simulink model "snb_b"  (R2012b)
settings: Solver=FixedStepDiscrete  SolverMode=SingleTasking  StartTime=0.0  StopTime=10000  RelTol=1e-3
undefined symbols (not defined in the file): Down, pfb_coeff_gen_calc, Up, xlipgetpartsetting
libraries: xbsIndex_r4 x14917, casper_library_misc x20, casper_library_communications x8, xps_library x3, casper_library_delays x3
(part 34 of 96)

== system snb_b/unpack_and_reorder/check_timestep_one ==
  note: The timestamp is only allowed to be smaller
      | than or equal to the last timestamp plus one.
  valid : Inport
  time : Inport  Port=2
  AddSub : xbsIndex_r4/AddSub  mode=Addition  use_carryin=off  use_carryout=off  en=off  latency=0  precision=Full  arith_type=Unsigned  n_bits=16  bin_pt=14  quantization=Truncate  overflow=Wrap  dbl_ovrd=off  use_behavioral_HDL=off  hw_selection=Fabric  pipelined=off  block_type=addsub
  Constant1 : xbsIndex_r4/Constant  const=1  gui_display_data_type=Fixed-point  arith_type=Unsigned  n_bits=1  bin_pt=0  preci_type=Single  exp_width=8  frac_width=24  explicit_period=on  period=1  equ=P=C  opselect=C  inp2=PCIN>>17  opr=+  inp1=P  carry=CIN  dbl_ovrd=off  block_type=constant
  Delay1 : xbsIndex_r4/Delay  rst=off  infoeditControl=Selection of Reset will increase slice count due to use of real FFs and instead of SRLs  en=off  latency=1  dbl_ovrd=off  reg_retiming=on  block_type=delay
  Delay2 : xbsIndex_r4/Delay  rst=off  infoeditControl=Selection of Reset will increase slice count due to use of real FFs and instead of SRLs  en=off  latency=1  dbl_ovrd=off  reg_retiming=on  block_type=delay
  Logical : xbsIndex_r4/Logical  logical_function=AND  inputs=2  en=off  latency=1  precision=Full  arith_type=Unsigned  n_bits=16  bin_pt=0  align_bp=on  dbl_ovrd=off  block_type=logical
  Logical1 : xbsIndex_r4/Logical  logical_function=AND  inputs=2  en=off  latency=1  precision=Full  arith_type=Unsigned  n_bits=16  bin_pt=0  align_bp=on  dbl_ovrd=off  block_type=logical
  Logical2 : xbsIndex_r4/Logical  logical_function=OR  inputs=2  en=off  latency=0  precision=Full  arith_type=Unsigned  n_bits=16  bin_pt=0  align_bp=on  dbl_ovrd=off  block_type=logical
  Register4 : xbsIndex_r4/Register  init=0  rst=off  en=on  dbl_ovrd=off  block_type=register
  Relational : xbsIndex_r4/Relational  mode=a>b  en=off  latency=1  dbl_ovrd=off  block_type=relational
  Relational1 : xbsIndex_r4/Relational  mode=a<=b  en=off  latency=1  dbl_ovrd=off  block_type=relational
  edge_detect : Subsystem  AncestorBlock=casper_library_misc/edge_detect  mask(edge_detect){edge=Rising, polarity=Active High, x_in=[0 0.08 0.08 0.16 0.16 0.24 0.24 0.32 0.32 0.4], y_in=[-1 -1  1  1  1  1  1  1  1  1], x_out=[0.6 0.68 0.68 0.76 0.76 0.84 0.84 0.92 0.92 1], y_out=[-1 -1  1  1 -1 -1 -1 -1 -1 -1]}
      mask prompts: edge "Edge Type"; polarity "Output Polarity"; x_in "Input X Positions"; y_in "Input Y Positions"; x_out "Output X Positions"; y_out "Output Y Positions"
      mask help: Output is active for one-cycle after each edge of the specified type (i.e. rising, falling or both).
      mask init: same as snb_b/edge_detect1
      settings: AttributesFormatString=|
      | rising edges
      | active high
      mask Help: Output is active for one-cycle after each edge of the specified type (i.e. rising, falling, or both).  Latency is zero.
      mask TypeOptions edge: Rising | Falling | Both
      mask TypeOptions polarity: Active High | Active Low
      mask Display:
      | plot(x_in_num,0.5+y_in_num*0.2);
      | plot(x_out_num,0.5+y_out_num*0.2);
  edge_detect1 : Subsystem  AncestorBlock=casper_library_misc/edge_detect  mask(edge_detect){edge=Rising, polarity=Active High, x_in=[0 0.08 0.08 0.16 0.16 0.24 0.24 0.32 0.32 0.4], y_in=[-1 -1  1  1  1  1  1  1  1  1], x_out=[0.6 0.68 0.68 0.76 0.76 0.84 0.84 0.92 0.92 1], y_out=[-1 -1  1  1 -1 -1 -1 -1 -1 -1]}
      mask prompts: edge "Edge Type"; polarity "Output Polarity"; x_in "Input X Positions"; y_in "Input Y Positions"; x_out "Output X Positions"; y_out "Output Y Positions"
      mask help: Output is active for one-cycle after each edge of the specified type (i.e. rising, falling or both).
      mask init: same as snb_b/edge_detect1
      settings: AttributesFormatString=|
      | rising edges
      | active high
      mask Help: Output is active for one-cycle after each edge of the specified type (i.e. rising, falling, or both).  Latency is zero.
      mask TypeOptions edge: Rising | Falling | Both
      mask TypeOptions polarity: Active High | Active Low
      mask Display:
      | plot(x_in_num,0.5+y_in_num*0.2);
      | plot(x_out_num,0.5+y_out_num*0.2);
  edge_detect2 : Subsystem  AncestorBlock=casper_library_misc/edge_detect  mask(edge_detect){edge=Rising, polarity=Active High, x_in=[0 0.08 0.08 0.16 0.16 0.24 0.24 0.32 0.32 0.4], y_in=[-1 -1  1  1  1  1  1  1  1  1], x_out=[0.6 0.68 0.68 0.76 0.76 0.84 0.84 0.92 0.92 1], y_out=[-1 -1  1  1 -1 -1 -1 -1 -1 -1]}
      mask prompts: edge "Edge Type"; polarity "Output Polarity"; x_in "Input X Positions"; y_in "Input Y Positions"; x_out "Output X Positions"; y_out "Output Y Positions"
      mask help: Output is active for one-cycle after each edge of the specified type (i.e. rising, falling or both).
      mask init: same as snb_b/edge_detect1
      settings: AttributesFormatString=|
      | rising edges
      | active high
      mask Help: Output is active for one-cycle after each edge of the specified type (i.e. rising, falling, or both).  Latency is zero.
      mask TypeOptions edge: Rising | Falling | Both
      mask TypeOptions polarity: Active High | Active Low
      mask Display:
      | plot(x_in_num,0.5+y_in_num*0.2);
      | plot(x_out_num,0.5+y_out_num*0.2);
  relock : Outport
  time_error_future : Outport  Port=2
  time_error_past : Outport  Port=3
  wires:
  AddSub/1 -> Relational/2  "lasttime+1"
  Register4/1 -> AddSub/2, Relational1/2  "lastime"
  Relational/1 -> Logical/1  "neq"
  edge_detect/1(out) -> Delay2/1, Delay1/1  "newpacket"
  valid/1 -> edge_detect/1(in)  "valid"
  Logical/1 -> edge_detect1/1(in)  "timestep_problem"
  Constant1/1 -> AddSub/1
  time/1 -> Relational/1, Relational1/1, Register4/1  "time"
  Delay1/1 -> Logical/2, Logical1/2
  Relational1/1 -> Logical1/1
  Logical1/1 -> edge_detect2/1(in)
  Delay2/1 -> Register4/2
  edge_detect1/1(out) -> Logical2/1, time_error_future/1
  edge_detect2/1(out) -> Logical2/2, time_error_past/1
  Logical2/1 -> relock/1

== system snb_b/unpack_and_reorder/digitiser_data_unpack1 ==
  start64 : Inport
  data64 : Inport  Port=2
  valid64 : Inport  Port=3
  eofi : Inport  Port=4
  misci : Inport  Port=5
  Concat : xbsIndex_r4/Concat  num_inputs=2  dbl_ovrd=off  block_type=concat
  bus_create7 : Subsystem  AncestorBlock=casper_library_flow_control/bus_create  mask(bus_create){inputNum=5}
      mask prompts: inputNum "Number of inputs:"
      mask init:
      | bus_create_init(gcb,...
      |     'inputNum', inputNum);
  eof : xbsIndex_r4/Slice  nbits=1  boolean_output=on  mode=Upper Bit Location + Width  bit1=0  base1=MSB of Input  bit0=0  base0=LSB of Input  dbl_ovrd=off  block_type=slice
  misc : xbsIndex_r4/Slice  nbits=1  boolean_output=off  mode=Two Bit Locations  bit1=-1  base1=MSB of Input  bit0=0  base0=LSB of Input  dbl_ovrd=off  block_type=slice
  unpack_64_to_1 : Subsystem
  dout80 : Outport
  eofo : Outport  Port=2
  dvalid80 : Outport  Port=3
  misco : Outport  Port=4
  start80 : Outport  Port=5
  all_debug : Outport  Port=6
  wires:
  misc/1 -> misco/1, bus_create7/5(in5)
  bus_create7/1(bus_out) -> all_debug/1
  start64/1 -> unpack_64_to_1/1(pkt_start)
  eof/1 -> eofo/1, bus_create7/4(in4)
  unpack_64_to_1/4(misco) -> eof/1, misc/1
  Concat/1 -> unpack_64_to_1/4(misci)
  misci/1 -> Concat/2
  data64/1 -> unpack_64_to_1/2(data64)
  unpack_64_to_1/1(start80) -> start80/1, bus_create7/1(in1)
  eofi/1 -> Concat/1
  unpack_64_to_1/3(valid80) -> dvalid80/1, bus_create7/2(in2)
  unpack_64_to_1/2(data80) -> dout80/1, bus_create7/3(in3)
  valid64/1 -> unpack_64_to_1/3(valid64)

== system snb_b/unpack_and_reorder/digitiser_data_unpack2 ==
  start64 : Inport
  data64 : Inport  Port=2
  valid64 : Inport  Port=3
  eofi : Inport  Port=4
  misci : Inport  Port=5
  Concat : xbsIndex_r4/Concat  num_inputs=2  dbl_ovrd=off  block_type=concat
  bus_create7 : Subsystem  AncestorBlock=casper_library_flow_control/bus_create  mask(bus_create){inputNum=5}
      mask prompts: inputNum "Number of inputs:"
      mask init:
      | bus_create_init(gcb,...
      |     'inputNum', inputNum);
  eof : xbsIndex_r4/Slice  nbits=1  boolean_output=on  mode=Upper Bit Location + Width  bit1=0  base1=MSB of Input  bit0=0  base0=LSB of Input  dbl_ovrd=off  block_type=slice
  misc : xbsIndex_r4/Slice  nbits=1  boolean_output=off  mode=Two Bit Locations  bit1=-1  base1=MSB of Input  bit0=0  base0=LSB of Input  dbl_ovrd=off  block_type=slice
  unpack_64_to_1 : Subsystem
  dout80 : Outport
  eofo : Outport  Port=2
  dvalid80 : Outport  Port=3
  misco : Outport  Port=4
  start80 : Outport  Port=5
  all_debug : Outport  Port=6
  wires:
  valid64/1 -> unpack_64_to_1/3(valid64)
  unpack_64_to_1/2(data80) -> bus_create7/3(in3), dout80/1
  unpack_64_to_1/3(valid80) -> bus_create7/2(in2), dvalid80/1
  eofi/1 -> Concat/1
  unpack_64_to_1/1(start80) -> bus_create7/1(in1), start80/1
  data64/1 -> unpack_64_to_1/2(data64)
  misci/1 -> Concat/2
  Concat/1 -> unpack_64_to_1/4(misci)
  unpack_64_to_1/4(misco) -> misc/1, eof/1
  eof/1 -> bus_create7/4(in4), eofo/1
  start64/1 -> unpack_64_to_1/1(pkt_start)
  bus_create7/1(bus_out) -> all_debug/1
  misc/1 -> bus_create7/5(in5), misco/1

== system snb_b/unpack_and_reorder/digitiser_data_unpack3 ==
  start64 : Inport
  data64 : Inport  Port=2
  valid64 : Inport  Port=3
  eofi : Inport  Port=4
  misci : Inport  Port=5
  Concat : xbsIndex_r4/Concat  num_inputs=2  dbl_ovrd=off  block_type=concat
  bus_create7 : Subsystem  AncestorBlock=casper_library_flow_control/bus_create  mask(bus_create){inputNum=5}
      mask prompts: inputNum "Number of inputs:"
      mask init:
      | bus_create_init(gcb,...
      |     'inputNum', inputNum);
  eof : xbsIndex_r4/Slice  nbits=1  boolean_output=on  mode=Upper Bit Location + Width  bit1=0  base1=MSB of Input  bit0=0  base0=LSB of Input  dbl_ovrd=off  block_type=slice
  misc : xbsIndex_r4/Slice  nbits=1  boolean_output=off  mode=Two Bit Locations  bit1=-1  base1=MSB of Input  bit0=0  base0=LSB of Input  dbl_ovrd=off  block_type=slice
  unpack_64_to_1 : Subsystem
  dout80 : Outport
  eofo : Outport  Port=2
  dvalid80 : Outport  Port=3
  misco : Outport  Port=4
  start80 : Outport  Port=5
  all_debug : Outport  Port=6
  wires:
  misc/1 -> misco/1, bus_create7/5(in5)
  bus_create7/1(bus_out) -> all_debug/1
  start64/1 -> unpack_64_to_1/1(pkt_start)
  eof/1 -> eofo/1, bus_create7/4(in4)
  unpack_64_to_1/4(misco) -> eof/1, misc/1
  Concat/1 -> unpack_64_to_1/4(misci)
  misci/1 -> Concat/2
  data64/1 -> unpack_64_to_1/2(data64)
  unpack_64_to_1/1(start80) -> start80/1, bus_create7/1(in1)
  eofi/1 -> Concat/1
  unpack_64_to_1/3(valid80) -> dvalid80/1, bus_create7/2(in2)
  unpack_64_to_1/2(data80) -> dout80/1, bus_create7/3(in3)
  valid64/1 -> unpack_64_to_1/3(valid64)

== system snb_b/unpack_and_reorder/digitiser_data_unpack4 ==
  start64 : Inport
  data64 : Inport  Port=2
  valid64 : Inport  Port=3
  eofi : Inport  Port=4
  misci : Inport  Port=5
  Concat : xbsIndex_r4/Concat  num_inputs=2  dbl_ovrd=off  block_type=concat
  bus_create7 : Subsystem  AncestorBlock=casper_library_flow_control/bus_create  mask(bus_create){inputNum=5}
      mask prompts: inputNum "Number of inputs:"
      mask init:
      | bus_create_init(gcb,...
      |     'inputNum', inputNum);
  eof : xbsIndex_r4/Slice  nbits=1  boolean_output=on  mode=Upper Bit Location + Width  bit1=0  base1=MSB of Input  bit0=0  base0=LSB of Input  dbl_ovrd=off  block_type=slice
  misc : xbsIndex_r4/Slice  nbits=1  boolean_output=off  mode=Two Bit Locations  bit1=-1  base1=MSB of Input  bit0=0  base0=LSB of Input  dbl_ovrd=off  block_type=slice
  unpack_64_to_1 : Subsystem
  dout80 : Outport
  eofo : Outport  Port=2
  dvalid80 : Outport  Port=3
  misco : Outport  Port=4
  start80 : Outport  Port=5
  all_debug : Outport  Port=6
  wires:
  valid64/1 -> unpack_64_to_1/3(valid64)
  unpack_64_to_1/2(data80) -> bus_create7/3(in3), dout80/1
  unpack_64_to_1/3(valid80) -> bus_create7/2(in2), dvalid80/1
  eofi/1 -> Concat/1
  unpack_64_to_1/1(start80) -> bus_create7/1(in1), start80/1
  data64/1 -> unpack_64_to_1/2(data64)
  misci/1 -> Concat/2
  Concat/1 -> unpack_64_to_1/4(misci)
  unpack_64_to_1/4(misco) -> misc/1, eof/1
  eof/1 -> bus_create7/4(in4), eofo/1
  start64/1 -> unpack_64_to_1/1(pkt_start)
  bus_create7/1(bus_out) -> all_debug/1
  misc/1 -> bus_create7/5(in5), misco/1

== system snb_b/unpack_and_reorder/din_expand ==
  bus_in : Inport
  reinterpret{1..4} (4 alike) : xbsIndex_r4/Reinterpret  force_arith_type=on  arith_type=Unsigned  force_bin_pt=on  bin_pt=0  block_type=reinterpret
  slice1 : xbsIndex_r4/Slice  nbits=64  boolean_output=off  mode=Upper Bit Location + Width  bit1=-192  base1=MSB of Input  bit0=0  base0=LSB of Input  dbl_ovrd=off  block_type=slice
  slice2 : xbsIndex_r4/Slice  nbits=64  boolean_output=off  mode=Upper Bit Location + Width  bit1=-128  base1=MSB of Input  bit0=0  base0=LSB of Input  dbl_ovrd=off  block_type=slice
  slice3 : xbsIndex_r4/Slice  nbits=64  boolean_output=off  mode=Upper Bit Location + Width  bit1=-64  base1=MSB of Input  bit0=0  base0=LSB of Input  dbl_ovrd=off  block_type=slice
  slice4 : xbsIndex_r4/Slice  nbits=64  boolean_output=off  mode=Upper Bit Location + Width  bit1=0  base1=MSB of Input  bit0=0  base0=LSB of Input  dbl_ovrd=off  block_type=slice
  msb_out4 : Outport
  out3 : Outport  Port=2
  out2 : Outport  Port=3
  lsb_out1 : Outport  Port=4
  wires:
  bus_in/1 -> slice4/1, slice3/1, slice2/1, slice1/1
  slice4/1 -> reinterpret4/1
  reinterpret4/1 -> msb_out4/1
  slice3/1 -> reinterpret3/1
  reinterpret3/1 -> out3/1
  slice2/1 -> reinterpret2/1
  reinterpret2/1 -> out2/1
  slice1/1 -> reinterpret1/1
  reinterpret1/1 -> lsb_out1/1

== system snb_b/unpack_and_reorder/en_expand ==
  bus_in : Inport
  slice1 : xbsIndex_r4/Slice  nbits=1  boolean_output=on  mode=Upper Bit Location + Width  bit1=-3  base1=MSB of Input  bit0=0  base0=LSB of Input  dbl_ovrd=off  block_type=slice
  slice2 : xbsIndex_r4/Slice  nbits=1  boolean_output=on  mode=Upper Bit Location + Width  bit1=-2  base1=MSB of Input  bit0=0  base0=LSB of Input  dbl_ovrd=off  block_type=slice
  slice3 : xbsIndex_r4/Slice  nbits=1  boolean_output=on  mode=Upper Bit Location + Width  bit1=-1  base1=MSB of Input  bit0=0  base0=LSB of Input  dbl_ovrd=off  block_type=slice
  slice4 : xbsIndex_r4/Slice  nbits=1  boolean_output=on  mode=Upper Bit Location + Width  bit1=0  base1=MSB of Input  bit0=0  base0=LSB of Input  dbl_ovrd=off  block_type=slice
  msb_out4 : Outport
  out3 : Outport  Port=2
  out2 : Outport  Port=3
  lsb_out1 : Outport  Port=4
  wires:
  bus_in/1 -> slice4/1, slice3/1, slice2/1, slice1/1
  slice4/1 -> msb_out4/1
  slice3/1 -> out3/1
  slice2/1 -> out2/1
  slice1/1 -> lsb_out1/1

== system snb_b/unpack_and_reorder/eof_expand ==
  bus_in : Inport
  slice1 : xbsIndex_r4/Slice  nbits=1  boolean_output=on  mode=Upper Bit Location + Width  bit1=-3  base1=MSB of Input  bit0=0  base0=LSB of Input  dbl_ovrd=off  block_type=slice
  slice2 : xbsIndex_r4/Slice  nbits=1  boolean_output=on  mode=Upper Bit Location + Width  bit1=-2  base1=MSB of Input  bit0=0  base0=LSB of Input  dbl_ovrd=off  block_type=slice
  slice3 : xbsIndex_r4/Slice  nbits=1  boolean_output=on  mode=Upper Bit Location + Width  bit1=-1  base1=MSB of Input  bit0=0  base0=LSB of Input  dbl_ovrd=off  block_type=slice
  slice4 : xbsIndex_r4/Slice  nbits=1  boolean_output=on  mode=Upper Bit Location + Width  bit1=0  base1=MSB of Input  bit0=0  base0=LSB of Input  dbl_ovrd=off  block_type=slice
  msb_out4 : Outport
  out3 : Outport  Port=2
  out2 : Outport  Port=3
  lsb_out1 : Outport  Port=4
  wires:
  bus_in/1 -> slice4/1, slice3/1, slice2/1, slice1/1
  slice4/1 -> msb_out4/1
  slice3/1 -> out3/1
  slice2/1 -> out2/1
  slice1/1 -> lsb_out1/1

== system snb_b/unpack_and_reorder/fifo0 ==
  note: change tlag
      | as last data
      |  word leaves
  note: count up on last item of packet,
      | count down as last word leaves,
      | leave as is if both
  note: clear discard on
      | last word of packet
  note: We have received a good packet if
      | 1. discard line is low for whole time
      | 2. eof is high
      | 3. rx word count is the expected
      | multiple
      | 4.  rx word count is less than the
      | maximum allowed
      | 5. not discarding current packet due
      | to packet limit reached
      | 6. en is high
  note: discard new packet
      | if packet count
      | indicates already
      | at max we can
      | store
  note: a fifo overflow should never happen
      | as extra packets are discarded
      | and packets that are too large
      | are also discarded.
      | Kept as a a sanity check
  note: The flag buffer stores the word count
      | and flag associated with each packet
      | received. This is used to extract the
      | correct number of words and tag
      | it appropriately on the way out
  note: we do not allow writes to the data buffer if we know
      | that we are going to discard the current packet
  note: We start off in reset and hold
      | reset high till the end of the first
      | packet we receive
  note: We are done transmitting if
      | we have reached the end
      | of the data, or are in reset
  rst : Inport
  din : Inport  Port=2
  eof : Inport  Port=3
  en : Inport  Port=4
  discard : Inport  Port=5
  flagi : Inport  Port=6
  tx : Inport  Port=7
  Constant : xbsIndex_r4/Constant  const=2^scale_factor_bits-1  gui_display_data_type=Fixed-point  arith_type=Unsigned  n_bits=scale_factor_bits  bin_pt=0  preci_type=Single  exp_width=8  frac_width=24  explicit_period=on  period=1  equ=P=C  opselect=C  inp2=PCIN>>17  opr=+  inp1=P  carry=CIN  dbl_ovrd=off  block_type=constant
  Constant1 : xbsIndex_r4/Constant  const=0  gui_display_data_type=Boolean  arith_type=Boolean  n_bits=scale_factor_bits  bin_pt=0  preci_type=Single  exp_width=8  frac_width=24  explicit_period=on  period=1  equ=P=C  opselect=C  inp2=PCIN>>17  opr=+  inp1=P  carry=CIN  dbl_ovrd=off  block_type=constant
  Delay{,1..5,7..14} (14 alike) : xbsIndex_r4/Delay  rst=off  infoeditControl=Selection of Reset will increase slice count due to use of real FFs and instead of SRLs  en=off  latency=1  dbl_ovrd=off  reg_retiming=on  block_type=delay
      settings: block_version=11.4
  Delay6 : xbsIndex_r4/Delay  rst=on  infoeditControl=Selection of Reset will increase slice count due to use of real FFs and instead of SRLs  en=on  latency=1  dbl_ovrd=off  reg_retiming=on  block_type=delay
  Gateway Out{,1..20} (21 alike) : xbsIndex_r4/Gateway Out  inherit_from_input=off  hdl_port=on  timing_constraint=None  locs_specified=off  LOCs={}  UseAsDAC=off  DACChannel='1'  block_type=gatewayout
  Inverter{1..6} (6 alike) : xbsIndex_r4/Inverter  en=off  latency=0  dbl_ovrd=off  block_type=inv
  Logical{,3,5,11} (4 alike) : xbsIndex_r4/Logical  logical_function=AND  inputs=2  en=off  latency=0  precision=Full  arith_type=Unsigned  n_bits=16  bin_pt=0  align_bp=on  dbl_ovrd=off  block_type=logical
      Logical11 settings: block_version=11.4
  Logical1 : xbsIndex_r4/Logical  logical_function=AND  inputs=3  en=off  latency=0  precision=Full  arith_type=Unsigned  n_bits=16  bin_pt=0  align_bp=on  dbl_ovrd=off  block_type=logical
  Logical2 : xbsIndex_r4/Logical  logical_function=AND  inputs=6  en=off  latency=1  precision=Full  arith_type=Unsigned  n_bits=16  bin_pt=0  align_bp=on  dbl_ovrd=off  block_type=logical
  Logical{4,7..9} (4 alike) : xbsIndex_r4/Logical  logical_function=OR  inputs=2  en=off  latency=0  precision=Full  arith_type=Unsigned  n_bits=16  bin_pt=0  align_bp=on  dbl_ovrd=off  block_type=logical
      Logical7 settings: block_version=11.4
      Logical8 settings: block_version=11.4
      Logical9 settings: block_version=11.4
  Logical6 : xbsIndex_r4/Logical  logical_function=XOR  inputs=2  en=off  latency=0  precision=Full  arith_type=Unsigned  n_bits=16  bin_pt=0  align_bp=on  dbl_ovrd=off  block_type=logical
      settings: block_version=11.4
  Relational : xbsIndex_r4/Relational  mode=a=b  en=off  latency=0  dbl_ovrd=off  block_type=relational
  Slice : xbsIndex_r4/Slice  nbits=input_word_count_bits - scale_factor_bits  boolean_output=off  mode=Upper Bit Location + Width  bit1=0  base1=MSB of Input  bit0=0  base0=LSB of Input  dbl_ovrd=off  block_type=slice
  Terminator : Terminator
  Terminator1 : Terminator
  concat1 : xbsIndex_r4/Concat  num_inputs=2  dbl_ovrd=off  block_type=concat
  data_buffer : Subsystem  mask{depth_bits=input_word_count_bits+n_bits_depth, scale_factor=2^scale_factor_bits, full_bits=1, n_bits_in=n_bits_din, bram_latency=bram_latency}
      mask prompts: depth_bits "depth (2^?)"; scale_factor "output width scale factor"; full_bits "number of bits in %full signal"; n_bits_in "word size (bits)"; bram_latency "BRAM latency"
  discard_reg : xbsIndex_r4/Register  init=0  rst=on  en=on  dbl_ovrd=off  block_type=register
  discarding : xbsIndex_r4/Delay  rst=on  infoeditControl=Selection of Reset will increase slice count due to use of real FFs and instead of SRLs  en=on  latency=1  dbl_ovrd=off  reg_retiming=on  block_type=delay
      settings: block_version=11.4
  edge_detect : Subsystem  AncestorBlock=casper_library_misc/edge_detect  mask(edge_detect){edge=Rising, polarity=Active High, x_in=[0 0.08 0.08 0.16 0.16 0.24 0.24 0.32 0.32 0.4], y_in=[-1 -1  1  1  1  1  1  1  1  1], x_out=[0.6 0.68 0.68 0.76 0.76 0.84 0.84 0.92 0.92 1], y_out=[-1 -1  1  1 -1 -1 -1 -1 -1 -1]}
      mask prompts: edge "Edge Type"; polarity "Output Polarity"; x_in "Input X Positions"; y_in "Input Y Positions"; x_out "Output X Positions"; y_out "Output Y Positions"
      mask help: Output is active for one-cycle after each edge of the specified type (i.e. rising, falling or both).
      mask init: same as snb_b/edge_detect1
      settings: AttributesFormatString=|
      | rising edges
      | active high
      mask Help: Output is active for one-cycle after each edge of the specified type (i.e. rising, falling, or both).  Latency is zero.
      mask TypeOptions edge: Rising | Falling | Both
      mask TypeOptions polarity: Active High | Active Low
      mask Display:
      | plot(x_in_num,0.5+y_in_num*0.2);
      | plot(x_out_num,0.5+y_out_num*0.2);
  edge_detect1 : Subsystem  AncestorBlock=casper_library_misc/edge_detect  mask(edge_detect){edge=Falling, polarity=Active High, x_in=[0 0.08 0.08 0.16 0.16 0.24 0.24 0.32 0.32 0.4], y_in=[-1 -1  1  1  1  1  1  1  1  1], x_out=[0.6 0.68 0.68 0.76 0.76 0.84 0.84 0.92 0.92 1], y_out=[-1 -1  1  1 -1 -1 -1 -1 -1 -1]}
      mask prompts: edge "Edge Type"; polarity "Output Polarity"; x_in "Input X Positions"; y_in "Input Y Positions"; x_out "Output X Positions"; y_out "Output Y Positions"
      mask help: Output is active for one-cycle after each edge of the specified type (i.e. rising, falling or both).
      mask init: same as snb_b/edge_detect1
      settings: AttributesFormatString=|
      | falling edges
      | active high
      mask Help: Output is active for one-cycle after each edge of the specified type (i.e. rising, falling, or both).  Latency is zero.
      mask TypeOptions edge: Rising | Falling | Both
      mask TypeOptions polarity: Active High | Active Low
      mask Display:
      | plot(x_in_num,0.5+y_in_num*0.2);
      | plot(x_out_num,0.5+y_out_num*0.2);
  edge_detect2 : Subsystem  AncestorBlock=casper_library_misc/edge_detect  mask(edge_detect){edge=Rising, polarity=Active High, x_in=[0 0.08 0.08 0.16 0.16 0.24 0.24 0.32 0.32 0.4], y_in=[-1 -1  1  1  1  1  1  1  1  1], x_out=[0.6 0.68 0.68 0.76 0.76 0.84 0.84 0.92 0.92 1], y_out=[-1 -1  1  1 -1 -1 -1 -1 -1 -1]}
      mask prompts: edge "Edge Type"; polarity "Output Polarity"; x_in "Input X Positions"; y_in "Input Y Positions"; x_out "Output X Positions"; y_out "Output Y Positions"
      mask help: Output is active for one-cycle after each edge of the specified type (i.e. rising, falling or both).
      mask init: same as snb_b/edge_detect1
      settings: AttributesFormatString=|
      | rising edges
      | active high
      mask Help: Output is active for one-cycle after each edge of the specified type (i.e. rising, falling, or both).  Latency is zero.
      mask TypeOptions edge: Rising | Falling | Both
      mask TypeOptions polarity: Active High | Active Low
      mask Display:
      | plot(x_in_num,0.5+y_in_num*0.2);
      | plot(x_out_num,0.5+y_out_num*0.2);
  flag : xbsIndex_r4/Slice  nbits=n_bits_flag  boolean_output=off  mode=Lower Bit Location + Width  bit1=0  base1=MSB of Input  bit0=0  base0=LSB of Input  dbl_ovrd=off  block_type=slice
  flag_buffer : xbsIndex_r4/Dual Port RAM  depth=2^n_bits_depth  initVector=zeros(1, 2^n_bits_depth)  distributed_mem=Distributed memory  init_a=0  init_b=0  rst_a=off  rst_b=off  en_a=off  en_b=off  latency=1  write_mode_A=Read After Write  write_mode_B=Read After Write  dbl_ovrd=off  optimize=Area  block_type=dpram
  input : Scope  NumInputPorts=9
      settings: YMin=0~0~-1~0~3.25836e+46~5e+45~0~0~-5  YMax=1.2e+22~1~1~1~3.60134e+46~1.2e+46~1~750~5  SaveName=ScopeData4
  logical1 : xbsIndex_r4/Relational  mode=a=b  en=off  latency=0  dbl_ovrd=off  block_type=relational
  logical2 : xbsIndex_r4/Relational  mode=a>b  en=off  latency=1  dbl_ovrd=off  block_type=relational
  logical3 : xbsIndex_r4/Relational  mode=a=b  en=off  latency=1  dbl_ovrd=off  block_type=relational
  lsbs_wc : xbsIndex_r4/Slice  nbits=scale_factor_bits  boolean_output=off  mode=Lower Bit Location + Width  bit1=0  base1=MSB of Input  bit0=0  base0=LSB of Input  dbl_ovrd=off  block_type=slice
  msb_wc : xbsIndex_r4/Slice  nbits=1  boolean_output=on  mode=Upper Bit Location + Width  bit1=0  base1=MSB of Input  bit0=0  base0=LSB of Input  dbl_ovrd=off  block_type=slice
  output : Scope  NumInputPorts=7
      settings: YMin=-1~-1~-1~-1~-1~-1~-5  YMax=1~1~1~1~1~1~5  SaveName=ScopeData5
  output1 : Scope  NumInputPorts=5
      settings: YMin=0~0~0~0~0  YMax=1~1~600~1~300  SaveName=ScopeData8
  packet_count : xbsIndex_r4/Counter  cnt_type=Free Running  cnt_to=Inf  operation=Up/Down  start_count=0  cnt_by_val=1  arith_type=Unsigned  n_bits=n_bits_depth  bin_pt=0  load_pin=off  rst=on  en=on  explicit_period=on  period=1  dbl_ovrd=off  use_behavioral_HDL=on  implementation=Fabric  block_type=counter
  rd_add : xbsIndex_r4/Counter  cnt_type=Free Running  cnt_to=Inf  operation=Up  start_count=0  cnt_by_val=1  arith_type=Unsigned  n_bits=n_bits_depth  bin_pt=0  load_pin=off  rst=on  en=on  explicit_period=on  period=1  dbl_ovrd=off  use_behavioral_HDL=on  implementation=Fabric  block_type=counter
      settings: block_version=11.4
  rst_reg : xbsIndex_r4/Register  init=1  rst=on  en=on  dbl_ovrd=off  block_type=register
  word_count : xbsIndex_r4/Slice  nbits=input_word_count_bits  boolean_output=off  mode=Upper Bit Location + Width  bit1=0  base1=MSB of Input  bit0=0  base0=LSB of Input  dbl_ovrd=off  block_type=slice
  word_count1 : xbsIndex_r4/Slice  nbits=input_word_count_bits  boolean_output=off  mode=Lower Bit Location + Width  bit1=0  base1=MSB of Input  bit0=0  base0=LSB of Input  dbl_ovrd=off  block_type=slice
  word_count_in : xbsIndex_r4/Counter  cnt_type=Free Running  cnt_to=inf  operation=Up  start_count=0  cnt_by_val=1  arith_type=Unsigned  n_bits=input_word_count_bits + 1  bin_pt=0  load_pin=off  rst=on  en=on  explicit_period=on  period=1  dbl_ovrd=off  use_behavioral_HDL=on  implementation=Fabric  block_type=counter
  word_count_out : xbsIndex_r4/Counter  cnt_type=Free Running  cnt_to=inf  operation=Up  start_count=0  cnt_by_val=1  arith_type=Unsigned  n_bits=input_word_count_bits - scale_factor_bits  bin_pt=0  load_pin=off  rst=on  en=on  explicit_period=on  period=1  dbl_ovrd=off  use_behavioral_HDL=on  implementation=Fabric  block_type=counter
  wr_addr : xbsIndex_r4/Counter  cnt_type=Free Running  cnt_to=Inf  operation=Up  start_count=0  cnt_by_val=1  arith_type=Unsigned  n_bits=n_bits_depth  bin_pt=0  load_pin=off  rst=on  en=on  explicit_period=on  period=1  dbl_ovrd=off  use_behavioral_HDL=on  implementation=Fabric  block_type=counter
      settings: block_version=11.4
  zero : xbsIndex_r4/Constant  const=0  gui_display_data_type=Fixed-point  arith_type=Unsigned  n_bits=n_bits_depth  bin_pt=0  preci_type=Single  exp_width=8  frac_width=24  explicit_period=on  period=1  equ=P=C  opselect=C  inp2=PCIN>>17  opr=+  inp1=P  carry=CIN  dbl_ovrd=off  block_type=constant
  zero1 : xbsIndex_r4/Constant  const=0  gui_display_data_type=Fixed-point  arith_type=Unsigned  n_bits=2  bin_pt=0  preci_type=Single  exp_width=8  frac_width=24  explicit_period=on  period=1  equ=P=C  opselect=C  inp2=PCIN>>17  opr=+  inp1=P  carry=CIN  dbl_ovrd=off  block_type=constant
  zero2 : xbsIndex_r4/Constant  const=0  gui_display_data_type=Fixed-point  arith_type=Unsigned  n_bits=2  bin_pt=0  preci_type=Single  exp_width=8  frac_width=24  explicit_period=on  period=1  equ=P=C  opselect=C  inp2=PCIN>>17  opr=+  inp1=P  carry=CIN  dbl_ovrd=off  block_type=constant
  zero3 : xbsIndex_r4/Constant  const=2^n_bits_depth-1  gui_display_data_type=Fixed-point  arith_type=Unsigned  n_bits=n_bits_depth  bin_pt=0  preci_type=Single  exp_width=8  frac_width=24  explicit_period=on  period=1  equ=P=C  opselect=C  inp2=PCIN>>17  opr=+  inp1=P  carry=CIN  dbl_ovrd=off  block_type=constant
  dout : Outport
  flago : Outport  Port=2
  dvalid : Outport  Port=3
  done : Outport  Port=4
  ready : Outport  Port=5
  fifo_of : Outport  Port=6
  discading : Outport  Port=7
  wires:
  [rst_in] -> Logical9/1
  Logical9/1 -> Logical11/1
  logical1/1 -> Logical9/2
  rst_reg/1 -> [rst_in]
  [eof] -> rst_reg/3
  Constant1/1 -> rst_reg/1
  rst/1 -> rst_reg/2
  zero3/1 -> logical3/2
  word_count1/1 -> Delay11/1
  edge_detect2/1(out) -> discading/1
  [discarding] -> Inverter6/1
  [word_max] -> Inverter5/1
  msb_wc/1 -> [word_max]
  Inverter6/1 -> Logical1/1
  Inverter5/1 -> Logical1/2
  Logical1/1 -> data_buffer/2(we)
  discard_reg/1 -> Logical8/1
  discard/1 -> Logical/2
  Inverter1/1 -> Logical2/5
  logical3/1 -> [pkt_max]
  Inverter4/1 -> Logical2/4
  Inverter2/1 -> Logical2/1
  Logical4/1 -> discarding/2
  [rst_in] -> Logical4/1
  [word_max] -> Inverter4/1
  lsbs_wc/1 -> Relational/2
  Constant/1 -> Relational/1
  discarding/1 -> [discarding], Inverter1/1
  Logical3/1 -> discarding/3, discarding/1
  [pkt_max] -> Logical3/1
  zero2/1 -> Gateway Out5/1
  zero1/1 -> Gateway Out4/1
  flag_buffer/1 -> Terminator1/1
  rd_add/1 -> flag_buffer/4
  [eof] -> Logical5/2
  Inverter3/1 -> Logical5/1
  Logical5/1 -> data_buffer/6(discard), edge_detect2/1(in)
  [good_eof] -> Gateway Out20/1
  Gateway Out20/1 -> input/9
  [good_eof] -> Inverter3/1
  [eof] -> data_buffer/5(eof)
  Logical2/1 -> [good_eof]
  Relational/1 -> Logical2/3
  Delay14/1 -> flag_buffer/3
  Gateway Out19/1 -> output/7
  [good_eof] -> Logical6/2
  Gateway Out18/1 -> output1/5
  [good_eof] -> packet_count/1
  Delay8/1 -> Gateway Out17/1
  word_count_in/1 -> word_count1/1, lsbs_wc/1, msb_wc/1
  Gateway Out8/1 -> output/2
  Gateway Out11/1 -> output/4
  Gateway Out12/1 -> output/5
  Gateway Out9/1 -> output/3
  Gateway Out7/1 -> output/1
  Gateway Out17/1 -> output/6
  eof/1 -> word_count_in/1, Logical4/2, Logical2/2, Logical7/2, Delay13/1
  Delay2/1 -> Gateway Out1/1, Logical1/3
  [tx] -> edge_detect/1(in)
  Gateway Out15/1 -> output1/2
  Gateway Out13/1 -> output1/4
  [done] -> Gateway Out13/1
  Gateway Out16/1 -> output1/3
  [input_count] -> Gateway Out16/1
  [tx] -> Gateway Out15/1
  Gateway Out14/1 -> output1/1
  [done] -> Gateway Out14/1
  Delay13/1 -> [eof]
  logical2/1 -> [ready], ready/1, Gateway Out12/1
  tx/1 -> Delay6/3, Delay6/1
  [tx] -> Logical11/2
  Delay12/1 -> Gateway Out11/1
  Logical11/1 -> [done]
  Delay11/1 -> concat1/1, Gateway Out10/1, [count_in]
  Gateway Out10/1 -> input/8
  Delay10/1 -> Gateway Out9/1
  Delay9/1 -> Gateway Out8/1
  Delay7/1 -> Gateway Out7/1
  [tx] -> Delay10/1
  [good_eof] -> Delay7/1
  [ready] -> Gateway Out6/1
  Gateway Out6/1 -> input/7
  Gateway Out5/1 -> input/6
  Gateway Out4/1 -> input/5
  Gateway Out3/1 -> input/4
  Gateway Out2/1 -> input/3
  Gateway Out1/1 -> input/2
  Gateway Out/1 -> input/1
  Logical6/1 -> packet_count/3, Delay8/1
  Logical8/1 -> Inverter2/1, Gateway Out2/1
  Logical7/1 -> discard_reg/2
  [rst_in] -> Logical7/1
  Delay4/1 -> dvalid/1, Gateway Out19/1
  edge_detect/1(out) -> Logical6/1
  [rst_in] -> packet_count/2
  packet_count/1 -> logical3/1, Delay12/1, logical2/1
  zero/1 -> logical2/2
  data_buffer/1(%full) -> Terminator/1
  edge_detect1/1(out) -> rd_add/2, done/1
  Slice/1 -> logical1/2
  word_count_out/1 -> Gateway Out18/1, Delay9/1, logical1/1
  [input_count] -> Slice/1
  word_count/1 -> [input_count]
  flag/1 -> flago/1
  flag_buffer/2 -> word_count/1, flag/1
  Delay/1 -> concat1/2
  [done] -> word_count_out/1
  concat1/1 -> flag_buffer/2
  flagi/1 -> Delay/1
  [good_eof] -> wr_addr/2
  Delay5/1 -> fifo_of/1
  Delay3/1 -> dout/1
  [done] -> Delay6/2
  Delay1/1 -> Gateway Out/1, data_buffer/3(din)
  [tx] -> data_buffer/4(re)
  Delay6/1 -> [tx], word_count_out/2
  data_buffer/3(dout) -> Delay3/1
  data_buffer/2(of) -> Delay5/1
  [rst_in] -> wr_addr/1
  din/1 -> Delay1/1
  [rst_in] -> data_buffer/1(rst_rx)
  en/1 -> Delay2/1, Logical/1, Logical3/2, word_count_in/2, Delay14/1, Logical2/6
  wr_addr/1 -> flag_buffer/1, Gateway Out3/1
  data_buffer/4(dvalid) -> edge_detect1/1(in), Delay4/1
  [rst_in] -> rd_add/1
  Logical/1 -> discard_reg/1, discard_reg/3, Logical8/2
